simulink model "Key"  (R2020b)
settings: configuration reference "cs_ert" (kept outside this file)
settings Model: DataDictionary=Key.sldd  EnableAccessToBaseWorkspace=off  Creator=zhoutinglin  LastModifiedBy=zhoutinglin
settings ConfigSetRef: SourceName=cs_ert

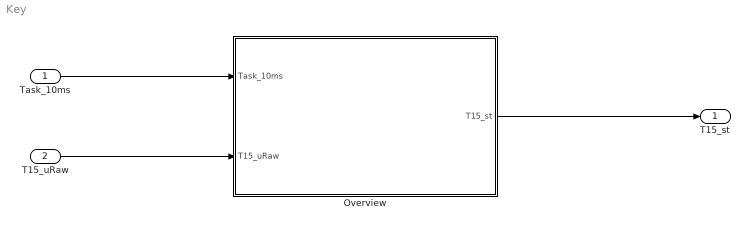
== system Key ==
  Task_10ms : Inport  OutputFunctionCall=on
  T15_uRaw : Inport  Port=2
  Overview : Subsystem
  T15_st : Outport
  wires:
  Task_10ms/1 -> Overview/1(Task_10ms)
  T15_uRaw/1 -> Overview/2(T15_uRaw)
  Overview/1(T15_st) -> T15_st/1

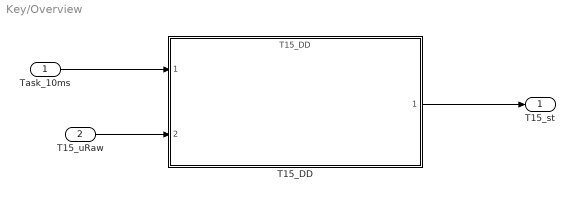
== system Key/Overview ==
  Task_10ms : Inport
  T15_uRaw : Inport  Port=2
  T15_DD : ModelReference  ModelNameDialog=T15_DD  SimulationMode=Normal  ScheduleRates=on  ModelReferenceVersion=6.2
  T15_st : Outport  VectorParamsAs1DForOutWhenUnconnected=off
  wires:
  T15_DD/1 -> T15_st/1
  T15_uRaw/1 -> T15_DD/2
  Task_10ms/1 -> T15_DD/1
